simulink model "quadRotorSim1"  (R2014a)
settings: Solver=FixedStepDiscrete  StartTime=0.0  StopTime=inf  FixedStep=dt  RelTol=1e-3
InitFcn:
  | DroneSimulation;
values from neighbouring files (symbols this model uses):
  angle_d1 = pi/2    (= 1.57079632679)    [DroneSimulation.m]
  d = scale*1.78    (= 1.78)    [DroneSimulation.m]
  d1 = scale*3.0    (= 3)    [DroneSimulation.m]
  dt = 2e-3    (= 0.002)    [DroneSimulation.m]
  L = scale*6.5    (= 6.5)    [DroneSimulation.m]
  l = scale*5    (= 5)    [DroneSimulation.m]
  orgn_d1 = [0;0; 8.6;]    [DroneSimulation.m]
  radiusAvatar = .2    (= 0.2)    [DroneSimulation.m]
  t_haplet = dt    (= 0.002)    [DroneSimulation.m]
undefined symbols (not defined in the file or in its folder): Cuav_d, Cvw_uav, navSphere, Obstacles, originOffset, Serial_Port, Standard_Devices
libraries: simulink x3, rtwinlib x2, vrlib x1
settings Model: SimulationMode=external  Creator=moriarty-admin  LastModifiedBy=moriarty-admin
settings DataIOCC: MaxDataPoints=20000
settings HardwareCC: ProdIntDivRoundTo=Zero  ProdEndianess=LittleEndian  ProdHWDeviceType=Generic->32-bit x86 compatible
settings RTWCC: SystemTargetFile=rtwin.tlc  TemplateMakefile=rtwin.tmf  Description=Real-Time Windows Target  ProcessScript=rtwin_make_rtw_hook  RTWCompilerOptimization=On
settings CodeAppCC: MaxIdLength=95
settings RTWinTargetCC: TargetLibSuffix=_rtwin.lib  TargetPreCompLibLocation=C:\Program Files\MATLAB\R2014a\toolbox\rtw\targets\rtwin\lib\win64

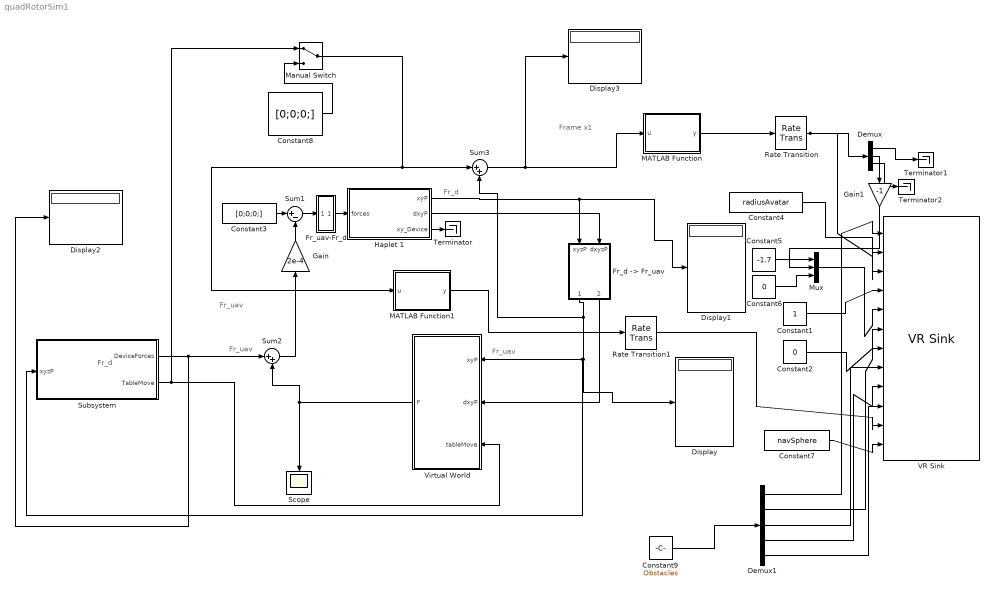
== system quadRotorSim1 ==
  note: Fr_uav
  note: Fr_uav
  note: Fr_uav
  note: Fr_d
  note: Fr_d
  note: Frame x1
  Constant1 : Constant  OutDataTypeStr=double
  Constant2 : Constant  Value=0  OutDataTypeStr=double
  Constant3 : Constant  Value=[0;0;0;]  OutDataTypeStr=double
  Constant4 : Constant  Value=radiusAvatar  OutDataTypeStr=double
  Constant5 : Constant  Value=-1.7  OutDataTypeStr=double
  Constant6 : Constant  Value=0  OutDataTypeStr=double
  Constant7 : Constant  Value=navSphere  OutDataTypeStr=double  SampleTime=-1
  Constant8 : Constant  Value=[0;0;0;]
  Constant9 : Constant  Value=Obstacles
  Demux : Demux  Outputs=3
  Demux1 : Demux  Outputs=[3 3 1 3 1]
  Display{,1..3} (4 alike) : Display
  "Fr_d -> Fr_uav" : MATLAB Function  TreatAsAtomicUnit=on
  Fr_uav-Fr_d : MATLAB Function  TreatAsAtomicUnit=on
  Gain : Gain  Gain=2e-4
  Gain1 : Gain  Gain=-1
  Haplet 1 : Subsystem
  MATLAB Function : MATLAB Function  TreatAsAtomicUnit=on
  MATLAB Function1 : MATLAB Function  TreatAsAtomicUnit=on
  Manual Switch : ManualSwitch
  Mux : Mux  Inputs=3
  Rate Transition : RateTransition  OutPortSampleTime=.02
  Rate Transition1 : RateTransition  OutPortSampleTime=.02
  Scope : Scope
      settings: YMin=-3250  YMax=1750  SaveName=ScopeData2
  Subsystem : Subsystem
  Sum1 : Sum  Inputs=|+-
  Sum2 : Sum  Inputs=|++
  Sum3 : Sum  Inputs=|++
  Terminator : Terminator
  Terminator1 : Terminator
  Terminator2 : Terminator
  VR Sink : vrlib/VR Sink  InstantiateOnLoad=on  SampleTime=-1  ViewEnable=on  RemoteChange=off  RemoteView=off  FieldsWritten=Wall.translation.3.1.1.double#Drone.translation.3.1.1.double#NavSphereRad.radius.1.1.1.double#DroneView.set_bind.1.1.1.logical#Shadow.translation.3.1.1.double#TopView.set_bind.1.1.1.logical#Cylinder1.translation.3.1.1.double#Obj_1_Cyl.radius.1.1.1.double#Cylinder2.translation.3.1.1.double#Obj_2_Cyl.radius.1.1.1.double#BigSphereTransform.translation.3.1.1.double#BigSphereRad.radius.1.1.1.double  WorldFileName=QuadWorld.wrl  AutoView=off  VideoDimensions=[]  AllowVariableSize=off  FigureProperties="{'Position', 'Name', 'Viewpoint', 'CameraBound', 'CameraDirection', 'CameraPosition', 'CameraUpVector', 'ZoomFactor', 'Antialiasing', 'Headlight', 'Lighting', 'NavPanel', 'StatusBar', 'ToolBar', 'Textures', 'Transparency', 'Triad', 'Wireframe', 'NavZones', 'NavMode', 'NavSpeed', 'CaptureFileFormat', 'CaptureFileName', 'Record2DCompressMethod', 'Record2DCompressQuality', 'Record2D', 'Record2DFileName', 'Record2DFPS'; [-1.6790000000000000e+03   1.0500000000000000e+02   1.6800000000000000e+03   9.2400000000000000e+02], '', 'DroneView', 'on', [-8.6047438598225434e-01   0.0000000000000000e+00  -5.0949370071526712e-01], [7.0183891575386017e+00   0.0000000000000000e+00   2.8232993930619337e+00], [0.0000000000000000e+00   1.0000000000000000e+00   0.0000000000000000e+00], [1.0000000000000000e+00], 'on', 'on', 'on', 'halfbar', 'on', 'on', 'on', 'on', 'none', 'off', 'off', 'walk', 'normal', 'tif', '%f_anim_%n.tif', 'auto', [7.5000000000000000e+01], 'off', '%f_anim_%n.avi', 'auto'}"
  Virtual World : Subsystem
  wires:
  Constant3/1 -> Sum1/1
  Sum1/1 -> Fr_uav-Fr_d/1(u)
  Gain/1 -> Sum1/2
  Virtual World/1(F) -> Scope/1, Sum2/2
  MATLAB Function/1(y) -> Rate Transition/1
  Sum3/1 -> Display3/1, MATLAB Function/1(u)
  Sum2/1 -> Gain/1
  Haplet 1/3(xy_Device) -> Terminator/1
  Subsystem/2(TableMove) -> Manual Switch/1, Virtual World/3(tableMove)
  Haplet 1/1(xyP) -> Display1/1, "Fr_d -> Fr_uav"/1(xyzP)
  "Fr_d -> Fr_uav"/1(xyzPout) -> Sum3/2, Display/1, Subsystem/1(xyzP), Virtual World/1(xyP)
  Fr_uav-Fr_d/1(y) -> Haplet 1/1(forces)
  Haplet 1/2(dxyP) -> "Fr_d -> Fr_uav"/2(dxyzP)
  "Fr_d -> Fr_uav"/2(dxyzPout) -> Virtual World/2(dxyP)
  Rate Transition/1 -> Demux/1, VR Sink/2
  Demux/1 -> Terminator1/1
  Demux/3 -> Terminator2/1
  Demux/2 -> Gain1/1
  Constant5/1 -> Mux/1
  Constant6/1 -> Mux/3
  Gain1/1 -> Mux/2
  MATLAB Function1/1(y) -> Rate Transition1/1
  Constant8/1 -> Manual Switch/2
  Manual Switch/1 -> Sum3/1, MATLAB Function1/1(u)
  Constant9/1 -> Demux1/1
  Demux1/3 -> VR Sink/8
  Demux1/5 -> VR Sink/10
  Subsystem/1(DeviceForces) -> Display2/1, Sum2/1
  Demux1/1 -> VR Sink/1
  Constant4/1 -> VR Sink/3
  Constant1/1 -> VR Sink/4
  Mux/1 -> VR Sink/5
  Constant2/1 -> VR Sink/6
  Demux1/2 -> VR Sink/7
  Demux1/4 -> VR Sink/9
  Rate Transition1/1 -> VR Sink/11
  Constant7/1 -> VR Sink/12

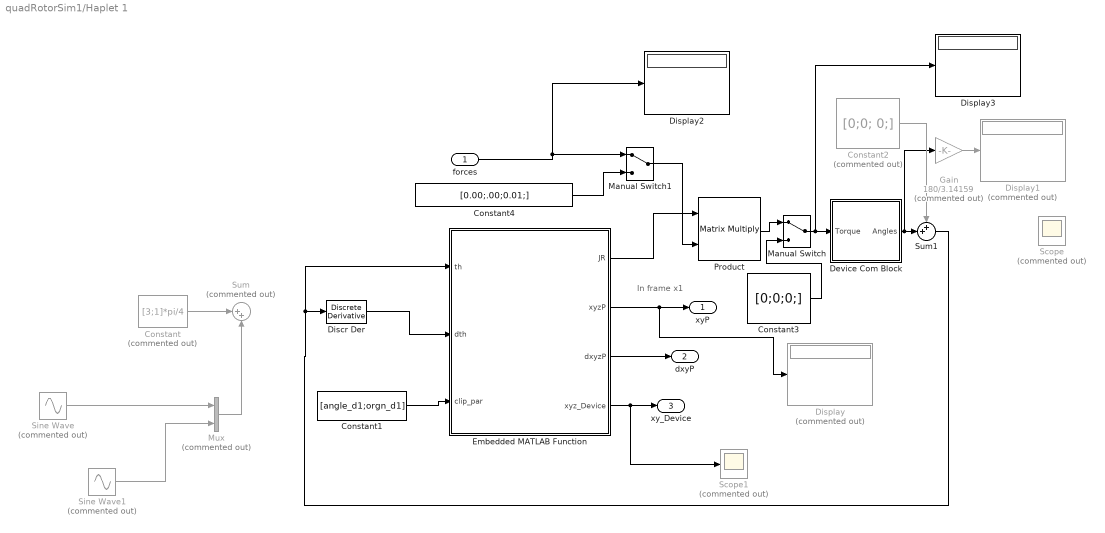
== system quadRotorSim1/Haplet 1 ==
  note: In frame x1
  forces : Inport
  Constant : Constant  Commented=on  Value=[3;1]*pi/4
  Constant1 : Constant  Value=[angle_d1;orgn_d1]
  Constant2 : Constant  Commented=on  Value=[0;0; 0;]
  Constant3 : Constant  Value=[0;0;0;]
  Constant4 : Constant  Value=[0.00;.00;0.01;]
  Device Com Block : Subsystem
  Discr Der : simulink/Discrete/Discrete Derivative  gainval=1.0  ICPrevScaledInput=[0;0;0;]  InputProcessing=Inherited  OutMin=[]  OutMax=[]  OutDataType=fixdt(1, 16)  OutScaling=2^-10  DoSatur=off
  Display : Display  Commented=on
  Display1 : Display  Commented=on
  Display2 : Display
  Display3 : Display
  Embedded MATLAB Function : MATLAB Function  TreatAsAtomicUnit=on
  Gain : Gain  Commented=on  Gain=180/3.14159
  Manual Switch : ManualSwitch
  Manual Switch1 : ManualSwitch
  Mux : Mux  Commented=on  Inputs=2
  Product : Product  Multiplication=Matrix(*)
  Scope : Scope  Commented=on
  Scope1 : Scope  Commented=on
      settings: YMax=8
  Sine Wave : Sin  Commented=on  Amplitude=pi/4  SampleTime=0.01
  Sine Wave1 : Sin  Commented=on  Amplitude=-pi/4  Phase=pi/6  SampleTime=0.01
  Sum : Sum  Commented=on  Inputs=|++
  Sum1 : Sum  Inputs=++|
  xyP : Outport
  dxyP : Outport  Port=2
  xy_Device : Outport  Port=3
  wires:
  Constant/1 -> Sum/1
  Sine Wave/1 -> Mux/1
  Mux/1 -> Sum/2
  Sine Wave1/1 -> Mux/2
  Discr Der/1 -> Embedded MATLAB Function/2(dth)
  Embedded MATLAB Function/2(xyzP) -> Display/1, xyP/1
  Embedded MATLAB Function/3(dxyzP) -> dxyP/1
  Embedded MATLAB Function/4(xyz_Device) -> Scope1/1, xy_Device/1
  Constant1/1 -> Embedded MATLAB Function/3(clip_par)
  forces/1 -> Manual Switch1/1, Display2/1
  Embedded MATLAB Function/1(JR) -> Product/1
  Device Com Block/1(Angles) -> Gain/1, Sum1/2
  Sum1/1 -> Embedded MATLAB Function/1(th), Discr Der/1
  Constant2/1 -> Sum1/1
  Manual Switch/1 -> Display3/1, Device Com Block/1(Torque)
  Product/1 -> Manual Switch/1
  Constant3/1 -> Manual Switch/2
  Gain/1 -> Display1/1
  Constant4/1 -> Manual Switch1/2
  Manual Switch1/1 -> Product/2

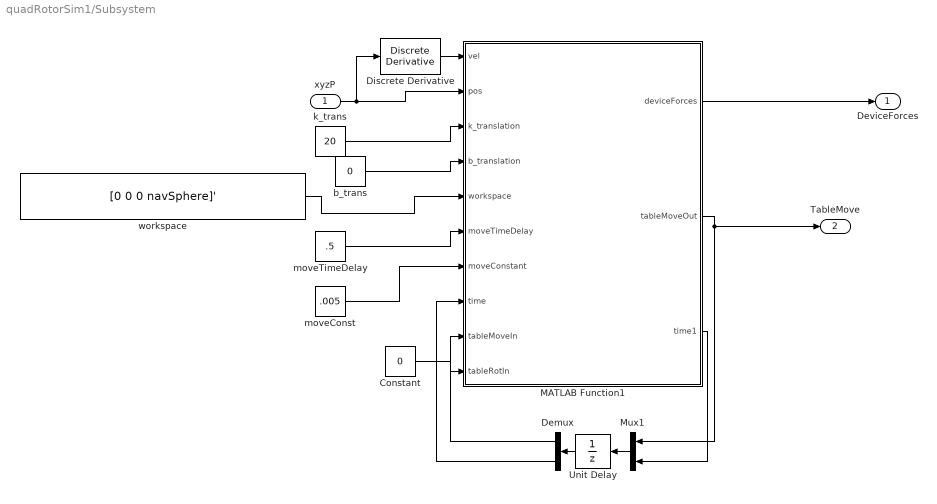
== system quadRotorSim1/Subsystem ==
  xyzP : Inport  PortDimensions=[1 3]  SampleTime=dt  Interpolate=off
  Constant : Constant  Value=0
  Demux : Demux  Outputs="[3  1]"
  Discrete Derivative : simulink/Discrete/Discrete Derivative  gainval=1.0  ICPrevScaledInput=0.0  InputProcessing=Inherited  OutMin=[]  OutMax=[]  OutDataType=fixdt(1, 16)  OutScaling=2^-10  DoSatur=off
  MATLAB Function1 : MATLAB Function  TreatAsAtomicUnit=on
  Mux1 : Mux  Inputs=[3 1 ]
  Unit Delay : UnitDelay  InitialCondition=[0 0 0 0]  SampleTime=-1
  b_trans : Constant  Value=0
  k_trans : Constant  Value=20
  moveConst : Constant  Value=.005
  moveTimeDelay : Constant  Value=.5
  workspace : Constant  Value=[0 0 0 navSphere]'
  DeviceForces : Outport
  TableMove : Outport  Port=2
  wires:
  MATLAB Function1/3(time1) -> Mux1/2
  Mux1/1 -> Unit Delay/1
  MATLAB Function1/1(deviceForces) -> DeviceForces/1
  k_trans/1 -> MATLAB Function1/3(k_translation)
  Unit Delay/1 -> Demux/1
  xyzP/1 -> Discrete Derivative/1, MATLAB Function1/2(pos)
  Demux/2 -> MATLAB Function1/8(time)
  moveConst/1 -> MATLAB Function1/7(moveConstant)
  Constant/1 -> MATLAB Function1/10(tableRotIn)
  moveTimeDelay/1 -> MATLAB Function1/6(moveTimeDelay)
  b_trans/1 -> MATLAB Function1/4(b_translation)
  Demux/1 -> MATLAB Function1/9(tableMoveIn)
  MATLAB Function1/2(tableMoveOut) -> TableMove/1, Mux1/1
  workspace/1 -> MATLAB Function1/5(workspace)
  Discrete Derivative/1 -> MATLAB Function1/1(vel)

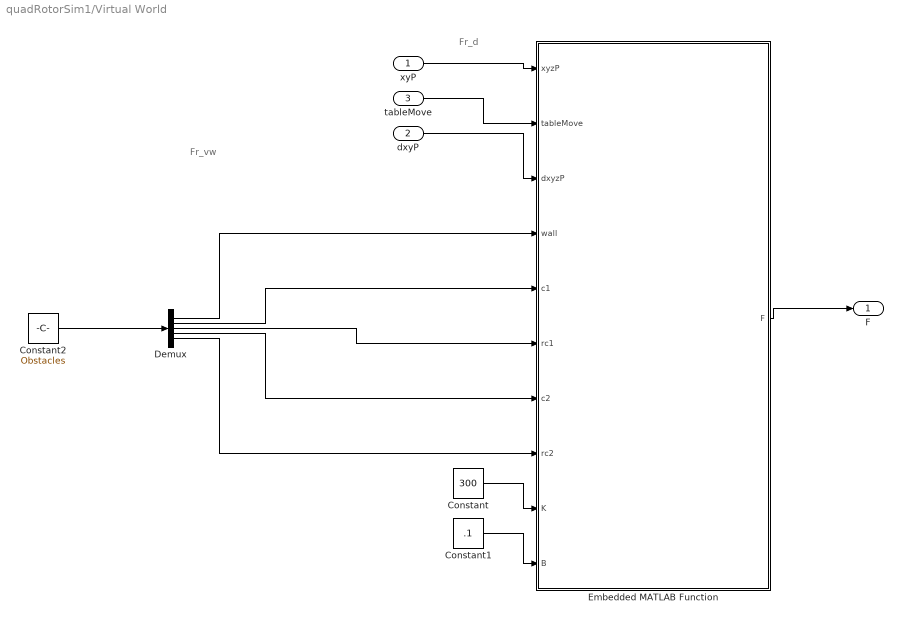
== system quadRotorSim1/Virtual World ==
  note: Fr_vw
  note: Fr_d
  xyP : Inport
  dxyP : Inport  Port=2
  tableMove : Inport  Port=3
  Constant : Constant  Value=300
  Constant1 : Constant  Value=.1
  Constant2 : Constant  Value=Obstacles
  Demux : Demux  Outputs=[3 3 1 3 1]
  Embedded MATLAB Function : MATLAB Function  TreatAsAtomicUnit=on
  F : Outport
  wires:
  xyP/1 -> Embedded MATLAB Function/1(xyzP)
  dxyP/1 -> Embedded MATLAB Function/3(dxyzP)
  Embedded MATLAB Function/1(F) -> F/1
  Constant/1 -> Embedded MATLAB Function/9(K)
  Constant1/1 -> Embedded MATLAB Function/10(B)
  tableMove/1 -> Embedded MATLAB Function/2(tableMove)
  Constant2/1 -> Demux/1
  Demux/3 -> Embedded MATLAB Function/6(rc1)
  Demux/2 -> Embedded MATLAB Function/5(c1)
  Demux/4 -> Embedded MATLAB Function/7(c2)
  Demux/1 -> Embedded MATLAB Function/4(wall)
  Demux/5 -> Embedded MATLAB Function/8(rc2)

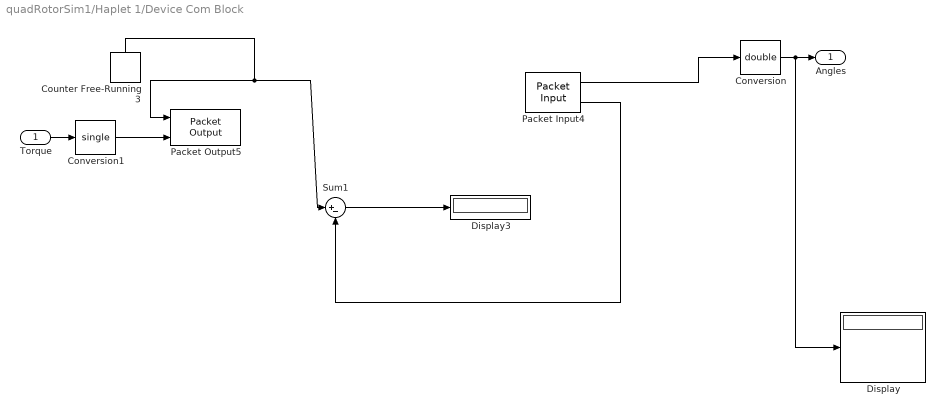
== system quadRotorSim1/Haplet 1/Device Com Block ==
  Torque : Inport
  Conversion : DataTypeConversion  OutDataTypeStr=double
  Conversion1 : DataTypeConversion  OutDataTypeStr=single
  Counter Free-Running3 : simulink/Sources/Counter Free-Running  NumBits=32  tsamp=t_haplet
  Display : Display
  Display3 : Display
  Packet Input4 : rtwinlib/Packet Input  SampleTime=t_haplet  MaxMissedTicks=inf  ShowMissedTicks=off  YieldWhenWaiting=on  DrvName=Standard_Devices/Serial_Port  DrvAddress=22  DrvOptions=[115200 8 0 0 0 0 0 0]  PacketSize=16  DataTypes={ '3*single';'uint32'}  ShowReady=off  ShowError=off  PacketID=1  ByteOrder=1  ShowTimestamp=off
      settings: AttributesFormatString=Standard Devices\nSerial Port [16h]
  Packet Output5 : rtwinlib/Packet Output  SampleTime=t_haplet  MaxMissedTicks=inf  ShowMissedTicks=off  YieldWhenWaiting=on  DrvName=Standard_Devices/Serial_Port  DrvAddress=22  DrvOptions=[115200 8 0 0 0 0 0 0]  PacketSize=16  DataTypes={'uint32'; '3*single'}  ShowReady=off  ShowError=off  PacketID=1  ByteOrder=1  InitialValue=[]  FinalValue=[]
      settings: AttributesFormatString=Standard Devices\nSerial Port [16h]
  Sum1 : Sum  Inputs=|+-
  Angles : Outport
  wires:
  Packet Input4/1 -> Conversion/1
  Packet Input4/2 -> Sum1/2
  Counter Free-Running3/1 -> Packet Output5/1, Sum1/1
  Sum1/1 -> Display3/1
  Torque/1 -> Conversion1/1
  Conversion1/1 -> Packet Output5/2
  Conversion/1 -> Display/1, Angles/1

== matlab function quadRotorSim1/Subsystem/MATLAB Function1 ==
  data: dt parameter; deviceForces output; vel input; pos input; k_translation input; b_translation input; workspace input; moveTimeDelay input; moveConstant input; time input; tableMoveIn input; tableMoveOut output; time1 output; tableRotIn input
function [deviceForces, tableMoveOut, time1] = fcn(dt, vel, pos, k_translation, b_translation, workspace, moveTimeDelay, moveConstant, time, tableMoveIn, tableRotIn)
% vel and pos are 3x1 vectors in cartesian coordinates

% workspace is a 6x1 vector with elements corresponding to x, y, z position
% of the center of the cylinder, the radius, the length of the cylinder,
% and the rotational limit

% device forces are 3x1, tableMove is 3x1 (w/ tableMove(2) = 0 since no y
% translation)


persistent clock;

if isempty(clock)
    clock = 0;
end

deviceForces = [0 0 0]';
tableMoveOut = tableMoveIn;
clock = clock + dt;

% pos_rad = sqrt((pos(1) - workspace(1))^2 + (pos(3) - workspace(3))^2);
x_diff= abs(pos(1)-workspace(1)); 
y_diff= abs(pos(2)-workspace(2)); 
z_diff= abs(pos(3)-workspace(3)); 

R=-[1 0 0; 0 1 0; 0 0 1; ]; 

if x_diff > workspace(4)
    
    deviceForces(1) = -k_translation*sign(pos(1) - workspace(1))*abs(x_diff - (workspace(4))) - b_translation*vel(1);
    
end

if y_diff > workspace(4)
    
    deviceForces(2) = -k_translation*sign(pos(2) - workspace(2))*abs(y_diff - (workspace(4))) - b_translation*vel(2);
    
end

if z_diff > workspace(4)
    
    deviceForces(3) = -k_translation*sign(pos(3) - workspace(3))*abs(z_diff - (workspace(4))) - b_translation*vel(3);
    
end


deviceForces(1:3)= R'*deviceForces(1:3); 


if x_diff < workspace(4) && y_diff < workspace(4) && z_diff < workspace(4)
    
    time1 = clock;
    
else
    
    time1 = time;
    
end
    
if (clock - time) > moveTimeDelay && x_diff > workspace(4)
    
    time1 = time;
    tableMoveOut(1) = tableMoveIn(1) + cos(tableRotIn)*moveConstant*sign(pos(1)-workspace(1))*(x_diff - workspace(4));
    tableMoveOut(2) = tableMoveIn(2) + sin(tableRotIn)*moveConstant*sign(pos(1)-workspace(1))*(x_diff - workspace(4));
    
    if (clock - time) > moveTimeDelay && y_diff > workspace(4)
    
        tableMoveOut(1) = tableMoveOut(1) - sin(tableRotIn)*moveConstant*sign(pos(2)-workspace(2))*(y_diff - workspace(4));
        tableMoveOut(2) = tableMoveOut(2) + cos(tableRotIn)*moveConstant*sign(pos(2)-workspace(2))*(y_diff - workspace(4));

    end
    
 
end  
      
    
if (clock - time) > moveTimeDelay && y_diff > workspace(4)
    
    time1 = time;
    tableMoveOut(1) = tableMoveIn(1) - sin(tableRotIn)*moveConstant*sign(pos(2)-workspace(2))*(y_diff - workspace(4));
    tableMoveOut(2) = tableMoveIn(2) + cos(tableRotIn)*moveConstant*sign(pos(2)-workspace(2))*(y_diff - workspace(4));

    if (clock - time) > moveTimeDelay && x_diff > workspace(4)
    
        tableMoveOut(1) = tableMoveOut(1) + cos(tableRotIn)*moveConstant*sign(pos(1)-workspace(1))*(x_diff - workspace(4));
        tableMoveOut(2) = tableMoveOut(2) + sin(tableRotIn)*moveConstant*sign(pos(1)-workspace(1))*(x_diff - workspace(4));
    end
    
end


if (clock - time) > moveTimeDelay && z_diff > workspace(4)

    tableMoveOut(3) = tableMoveOut(3) + moveConstant*sign(pos(3)-workspace(3))*(z_diff - workspace(4));
end

== matlab function quadRotorSim1/MATLAB Function ==
  data: u input; y output; Cvw_uav parameter
function y = fcn(u,Cvw_uav)
%#codegen

% R=[0 -1 0; 0 0 1; -1 0 0;]; 
y = Cvw_uav*u;

== matlab function quadRotorSim1/Virtual World/Embedded MATLAB Function ==
  data: F output; xyzP input; tableMove input; dxyzP input; wall input; c1 input; rc1 input; c2 input; rc2 input; K input; B input; radiusAvatar parameter; Cvw_uav parameter
function F  = EE_forces(xyzP, tableMove,dxyzP,wall,c1,rc1,c2,rc2,K,B,radiusAvatar,Cvw_uav)

% xyP,dxyP,xyC,dxyC,r_EE,r_B,K, scr_h, wallThickness,B_water, rho, g
% F=zeros(10,1); 
F=zeros(3,1);
% Xwall=-3; 
% Ywall=10; 
% Zwall=13;
% xyzC=[1; 7; 10.0]; 
% redBallRadius= 3;
% radiusAvatar=0.5; 
% K=150; 
% 
% B=0.035; 

% if xyzP(2)>Ywall; 
%     F=-K*[0;1;0]*(Ywall-xyzP(2))+ B*dxyzP;
% end
% 
%         
% if xyzP(3)>Zwall; 
%     F=-K*[0;0;1]*(Zwall-xyzP(3))+ B*dxyzP;
% elseif xyzP(3)<7; 
%     F=-K*[0;0;1]*(7-xyzP(3))+ B*dxyzP;
% end

Rot=Cvw_uav'; 

wall=Rot*wall-tableMove; 
floor=Rot*[0,0,0]'-tableMove; 
nwall=Rot*[0 0 1]'; 
nfloor=Rot*[0 1 0]'; 
c1=Rot*c1-tableMove; 
c2=Rot*c2-tableMove; 
vectW= xyzP-wall;
vectF= xyzP-floor; 
vect1= [xyzP(1:2)'-c1(1:2)' 0]';
vect2= [xyzP(1:2)'-c2(1:2)' 0]';
magW=norm(vectW,2); 
magF=norm(vectF,2); 
mag1=norm(vect1,2); 
mag2=norm(vect2,2); 


if dot(vectW, nwall)<radiusAvatar
    F=F-K*nwall*(radiusAvatar-dot(vectW, nwall))+B*dxyzP; 
end
if dot(vectF, nfloor)<radiusAvatar
    F=F-K*nfloor*(radiusAvatar-dot(vectF, nfloor))+B*dxyzP;   
end
if mag1<(rc1+radiusAvatar)
    F=F-K*vect1/mag1*((radiusAvatar+rc1)-mag1)+B*dxyzP; 
end
if mag2<(rc2+radiusAvatar) 
    F=F-K*vect2/mag2*((radiusAvatar+rc2)-mag2)+B*dxyzP; 
end

== matlab function quadRotorSim1/Fr_d -> Fr_uav ==
  data: xyzP input; dxyzP input; xyzPout output; Cuav_d parameter; dxyzPout output; originOffset parameter
function [xyzPout, dxyzPout] = fcn(xyzP, dxyzP,Cuav_d, originOffset)
%#codegen

% R=[0 -1 0; 0 0 1; -1 0 0;]; 
xyzPout = Cuav_d*(xyzP-originOffset');
dxyzPout = Cuav_d*dxyzP;

== matlab function quadRotorSim1/Fr_uav-Fr_d ==
  data: u input; y output; Cuav_d parameter
function y = fcn(u, Cuav_d)
%#codegen

% R=[0 -1 0; 0 0 1; -1 0 0;]; 
y = Cuav_d'*u;

== matlab function quadRotorSim1/MATLAB Function1 ==
  data: u input; y output; Cvw_uav parameter
function y = fcn(u,Cvw_uav)
%#codegen

% R=[0 -1 0; 0 0 1; -1 0 0;]; 
y = Cvw_uav*u+[0 .2 1.7]';

== matlab function quadRotorSim1/Haplet 1/Embedded MATLAB Function ==
  data: JR output; th input; dth input; l parameter; xyzP output; L parameter; d parameter; d1 parameter; dxyzP output; clip_par input; xyz_Device output
function [JR,xyzP,dxyzP,xyz_Device] = device_kin(th,dth,l,L,d,d1,clip_par)
%#codegen
% K is the stiffness of the plate
% Ks is the stiffness of the virtual spring in the first demo
% clip_par=[angle_d;orgn_d] specifies the angle and orgn at which the
% device is clipped on the screen

angle_d=clip_par(1);
orgn_d=[clip_par(2); clip_par(3); 7.9;];
c=cos(angle_d);
s=sin(angle_d);

[P,J,chain_points]=fwd_kin(th(1),th(2),-th(3),l,L,d,d1);
dxyzP=[c -s 0;s c 0; 0 0 1]*J*dth;                              % device to VW coords

P=[c -s 0;s c 0; 0 0 1]*P+orgn_d;
xyzP=P; 
% xyzP(2)=-xyzP(2);

for i=1:size(chain_points,1)
chain_points(i,:)=([c -s 0;s c 0; 0 0 1]*chain_points(i,:)'+orgn_d)';
end
xyz_Device=chain_points;

% J=J'; 
JR=J*[c s 0;-s c 0; 0 0 1];



function [EE,J,chain_points]=fwd_kin(th1,th2,th3, l,L,d,d1)

% some intermediate variables
c1=cos(th1);
c2=cos(th2);
s1=sin(th1);
s2=sin(th2);
xA=l*c1;yA=l*s1;
xB=d+l*c2;yB=l*s2;
R=xA^2+yA^2;
S=xB^2+yB^2;
M=(yA-yB)/(xB-xA);
N=0.5*(S-R)/(xB-xA);
a=M^2+1;
b=2*(M*N-M*xA-yA);
c=N^2-2*N*xA+R-L^2;
Delta=b^2-4*a*c;
Delta=Delta*(Delta>0);
y=(-b+sqrt(Delta))/(2*a); % +-
x=M*y+N;
phi1=angle((x-l*c1)/L+1i*(y-l*s1)/L);
phi2=angle((x-d-l*c2)/L+1i*(y-l*s2)/L);

c3=cos(th3); 
s3=sin(th3); 


R= [1 0 0; 0 c3 -s3; 0 s3 c3;]; 


% Points coordinates
EE= R*[x;y;d1;]; 

% Jacobian transposed calculations
Jpant=-l/sin(phi2-phi1)*[s1*sin(phi2-phi1)+sin(phi1)*sin(th1-phi2),-sin(phi1)*sin(th2-phi2);-c1*sin(phi2-phi1)-cos(phi1)*sin(th1-phi2),cos(phi1)*sin(th2-phi2)];

Q=[1 0; 0 c3; 0 s3;]; 
J3=[0; -s3*y-c3*d1; c3*y-s3*d1;]; 

J=[Q*Jpant', J3]'; 


% chain_points=[0;l*exp(1i*th1);E;d+l*exp(1i*th2);d];


origin1= R*[0;0;d1;]; 
link1=R*[xA; yA; d1;]; 
link2=R*[xB; yB; d1;]; 
origin2= R*[d;0;d1];     

chain_points= [origin1'; link1'; EE'; link2'; origin2';];
